simulink model "ethercat_v_1_0"  (R2016a)
settings: Solver=FixedStepDiscrete  StartTime=0.0  StopTime=inf  FixedStep=0.001  RelTol=1e-3
undefined symbols (not defined in the file): Hip_HAA
libraries: xpcethercatlib x16
settings Model: SimulationMode=external  Creator=Projectmarch  LastModifiedBy=Projectmarch
settings SolverCC: EnableConcurrentExecution=on
settings DataIOCC: SaveFormat=StructureWithTime
settings OptimizationCC: BlockReduction=off  OptimizeBlockIOStorage=off  BufferReuse=off  GlobalBufferReuse=off  ExpressionFolding=off  LocalBlockOutputs=off
settings HardwareCC: ProdBitPerPointer=32  ProdLargestAtomicFloat=None  ProdWordSize=32  ProdLongLongMode=on  ProdHWDeviceType=Generic->32-bit x86 compatible
settings RTWCC: SystemTargetFile=slrt.tlc  TemplateMakefile=slrt_default_tmf  Description=Simulink Real-Time  RTWCompilerOptimization=on

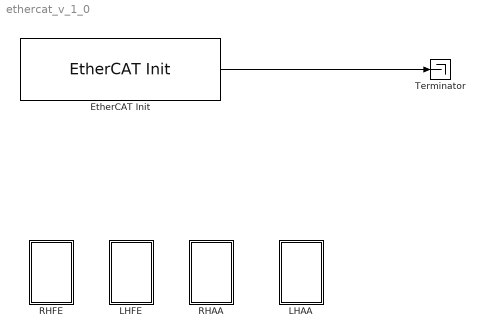
== system ethercat_v_1_0 ==
  "EtherCAT Init " : xpcethercatlib/EtherCAT Init   Priority=0  config_file=D:\Software\MATLAB\simulink-models\EtherCAT Config files\full_setup_v1.0.xml  device_id=0  pci_bus=2  pci_slot=0  dctuning=0  enaDebug=off  enaDC=on  errLink=off  masterDbg=off  stateChgDbg=off  baseClock=off  masterCfg=off  logFile='c:\dbglog.txt'  sample_time=0.001000
  LHAA : Subsystem
  LHFE : Subsystem
  RHAA : Subsystem
  RHFE : Subsystem
  Terminator : Terminator
  wires:
  "EtherCAT Init "/1 -> Terminator/1

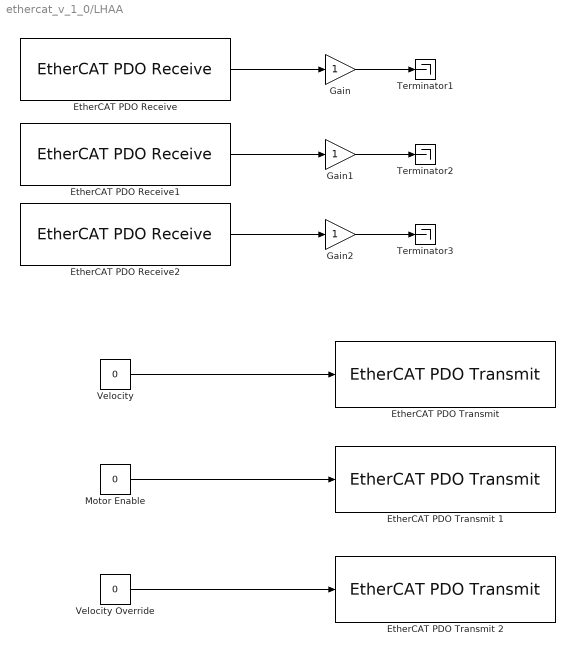
== system ethercat_v_1_0/LHAA ==
  EtherCAT PDO Receive : xpcethercatlib/EtherCAT PDO Receive  Priority=2  sig_name=Hip_HAA.Inputs.L_jointAngle  sig_offset=208  sig_type=uint32  type_size=32  sig_dim=1  device_id=0  sample_time=0.001000
  EtherCAT PDO Receive1 : xpcethercatlib/EtherCAT PDO Receive  Priority=2  sig_name=Hip_HAA.Inputs.L_motorAngle  sig_offset=272  sig_type=uint16  type_size=16  sig_dim=1  device_id=0  sample_time=0.001000
  EtherCAT PDO Receive2 : xpcethercatlib/EtherCAT PDO Receive  Priority=2  sig_name=Hip_HAA.Inputs.L_springAngle  sig_offset=240  sig_type=uint32  type_size=32  sig_dim=1  device_id=0  sample_time=0.001000
  "EtherCAT PDO Transmit " : xpcethercatlib/EtherCAT PDO Transmit   Priority=3  sig_name=Hip_HAA.Outputs.L_velocitySetPoint  sig_offset=208  sig_type=int16  type_size=16  sig_dim=1  device_id=0  sample_time=0.001000
  EtherCAT PDO Transmit 1 : xpcethercatlib/EtherCAT PDO Transmit   Priority=3  sig_name=Hip_HAA.Outputs.L_motorEnable  sig_offset=256  sig_type=uint8  type_size=8  sig_dim=1  device_id=0  sample_time=0.001000
  EtherCAT PDO Transmit 2 : xpcethercatlib/EtherCAT PDO Transmit   Priority=3  sig_name=Hip_HAA.Outputs.L_data[4]  sig_offset=480  sig_type=int32  type_size=32  sig_dim=1  device_id=0  sample_time=0.001000
  Gain : Gain
  Gain1 : Gain
  Gain2 : Gain
  Motor Enable : Constant  Value=0  OutDataTypeStr=uint8
  Terminator1 : Terminator
  Terminator2 : Terminator
  Terminator3 : Terminator
  Velocity : Constant  Value=0  OutDataTypeStr=int16
  Velocity Override : Constant  Value=0  OutDataTypeStr=int32
  wires:
  EtherCAT PDO Receive/1 -> Gain/1
  Gain1/1 -> Terminator2/1
  Gain/1 -> Terminator1/1
  Gain2/1 -> Terminator3/1
  EtherCAT PDO Receive1/1 -> Gain1/1
  EtherCAT PDO Receive2/1 -> Gain2/1
  Velocity/1 -> "EtherCAT PDO Transmit "/1
  Motor Enable/1 -> EtherCAT PDO Transmit 1/1
  Velocity Override/1 -> EtherCAT PDO Transmit 2/1

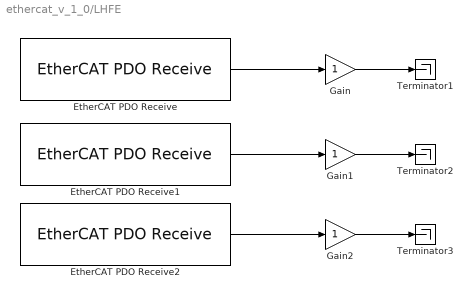
== system ethercat_v_1_0/LHFE ==
  EtherCAT PDO Receive : xpcethercatlib/EtherCAT PDO Receive  Priority=2  sig_name=Left_Leg.Inputs.H_jointAngle  sig_offset=1144  sig_type=uint32  type_size=32  sig_dim=1  device_id=0  sample_time=0.001000
  EtherCAT PDO Receive1 : xpcethercatlib/EtherCAT PDO Receive  Priority=2  sig_name=Left_Leg.Inputs.H_motorAngle  sig_offset=1208  sig_type=uint16  type_size=16  sig_dim=1  device_id=0  sample_time=0.001000
  EtherCAT PDO Receive2 : xpcethercatlib/EtherCAT PDO Receive  Priority=2  sig_name=Left_Leg.Inputs.H_springAngle  sig_offset=1176  sig_type=uint32  type_size=32  sig_dim=1  device_id=0  sample_time=0.001000
  Gain : Gain
  Gain1 : Gain
  Gain2 : Gain
  Terminator1 : Terminator
  Terminator2 : Terminator
  Terminator3 : Terminator
  wires:
  EtherCAT PDO Receive/1 -> Gain/1
  Gain1/1 -> Terminator2/1
  Gain/1 -> Terminator1/1
  Gain2/1 -> Terminator3/1
  EtherCAT PDO Receive1/1 -> Gain1/1
  EtherCAT PDO Receive2/1 -> Gain2/1

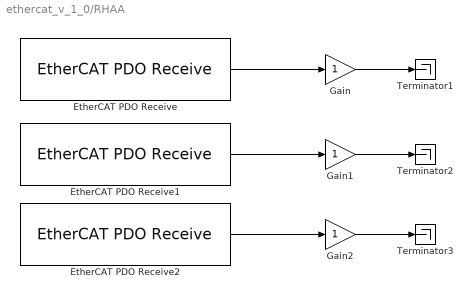
== system ethercat_v_1_0/RHAA ==
  EtherCAT PDO Receive : xpcethercatlib/EtherCAT PDO Receive  Priority=2  sig_name=Hip_HAA.Inputs.R_jointAngle  sig_offset=688  sig_type=uint32  type_size=32  sig_dim=1  device_id=0  sample_time=0.001000
  EtherCAT PDO Receive1 : xpcethercatlib/EtherCAT PDO Receive  Priority=2  sig_name=Hip_HAA.Inputs.R_motorAngle  sig_offset=752  sig_type=uint16  type_size=16  sig_dim=1  device_id=0  sample_time=0.001000
  EtherCAT PDO Receive2 : xpcethercatlib/EtherCAT PDO Receive  Priority=2  sig_name=Hip_HAA.Inputs.R_springAngle  sig_offset=720  sig_type=uint32  type_size=32  sig_dim=1  device_id=0  sample_time=0.001000
  Gain : Gain
  Gain1 : Gain
  Gain2 : Gain
  Terminator1 : Terminator
  Terminator2 : Terminator
  Terminator3 : Terminator
  wires:
  EtherCAT PDO Receive/1 -> Gain/1
  Gain1/1 -> Terminator2/1
  Gain/1 -> Terminator1/1
  Gain2/1 -> Terminator3/1
  EtherCAT PDO Receive1/1 -> Gain1/1
  EtherCAT PDO Receive2/1 -> Gain2/1

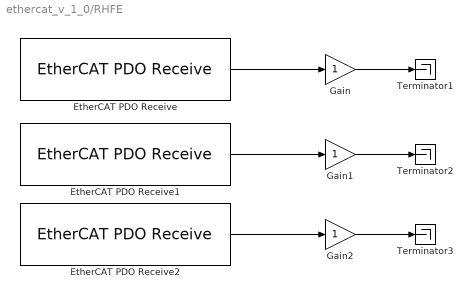
== system ethercat_v_1_0/RHFE ==
  EtherCAT PDO Receive : xpcethercatlib/EtherCAT PDO Receive  Priority=2  sig_name=Right_Leg.Inputs.H_jointAngle  sig_offset=1832  sig_type=uint32  type_size=32  sig_dim=1  device_id=0  sample_time=0.001000
  EtherCAT PDO Receive1 : xpcethercatlib/EtherCAT PDO Receive  Priority=2  sig_name=Right_Leg.Inputs.H_motorAngle  sig_offset=1896  sig_type=uint16  type_size=16  sig_dim=1  device_id=0  sample_time=0.001000
  EtherCAT PDO Receive2 : xpcethercatlib/EtherCAT PDO Receive  Priority=2  sig_name=Right_Leg.Inputs.H_springAngle  sig_offset=1864  sig_type=uint32  type_size=32  sig_dim=1  device_id=0  sample_time=0.001000
  Gain : Gain
  Gain1 : Gain
  Gain2 : Gain
  Terminator1 : Terminator
  Terminator2 : Terminator
  Terminator3 : Terminator
  wires:
  EtherCAT PDO Receive/1 -> Gain/1
  Gain1/1 -> Terminator2/1
  Gain/1 -> Terminator1/1
  Gain2/1 -> Terminator3/1
  EtherCAT PDO Receive1/1 -> Gain1/1
  EtherCAT PDO Receive2/1 -> Gain2/1
